simulink model "Delay3"  (R2017b)
settings: Solver=FixedStepDiscrete  StartTime=0.0  StopTime=10.0  FixedStep=0.200000  RelTol=1e-3  EnableMultiTasking=on
settings Model: Creator=hbourbou  LastModifiedBy=hbourbou
settings DataIOCC: LimitDataPoints=on  SaveFormat=Structure
settings OptimizationCC: LifeSpan=inf
settings DebuggingCC: SFUnexpectedBacktrackingDiag=warning  SFNoUnconditionalDefaultTransitionDiag=warning  SFExecutionAtInitializationDiag=none
settings HardwareCC: ProdBitPerPointer=32  ProdBitPerSizeT=32  ProdBitPerPtrDiffT=32  ProdLargestAtomicFloat=None  ProdIntDivRoundTo=Undefined  ProdEndianess=Unspecified  ProdWordSize=32  ProdHWDeviceType=32-bit Generic
settings ModelReferenceCC: PropagateSignalLabelsOutOfModel=off
settings CodeAppCC: StateflowObjectComments=on
settings GRTTargetCC: TargetLangStandard=C89/C90 (ANSI)  GeneratePreprocessorConditionals=Disable all
settings ConfigComp: CovMetricSettings=dw  CovHtmlReporting=on  CovSaveCumulativeToWorkspaceVar=on  CovSaveSingleToWorkspaceVar=on  CovExternalEMLEnable=off

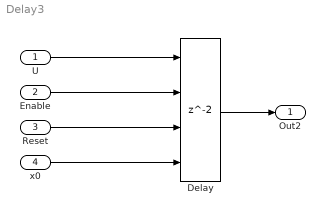
== system Delay3 ==
  U : Inport  PortDimensions=2
  Enable : Inport  Port=2  PortDimensions=1
  Reset : Inport  Port=3  OutDataTypeStr=boolean  PortDimensions=1
  x0 : Inport  Port=4
  Delay : Delay  InitialConditionSource=Input port  ExternalReset=Falling  ShowEnablePort=on
      settings: InputPortMap=u0,e6,r5,p4
  Out2 : Outport
  wires:
  Delay/1 -> Out2/1
  Enable/1 -> Delay/2
  Reset/1 -> Delay/3
  x0/1 -> Delay/4
  U/1 -> Delay/1
